simulink model "RT_Klausur_2011_A1"  (R2013a)
settings: Solver=ode45  StartTime=0.0  StopTime=10.0  RelTol=1e-3
values from neighbouring files (symbols this model uses):
  k = 1    [RT_Klausur_SS2014.m]    (also in RT_ctrl_analyse_proc.m = 5; RT_dennis_draussen.m = 50; RT_klausurvorb.m = 0.2; RT_lab_paramLead.m)
settings Model: Creator=mainster  LastModifiedBy=mainster

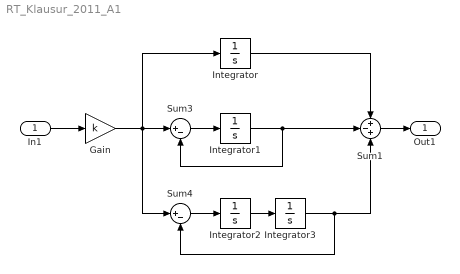
== system RT_Klausur_2011_A1 ==
  In1 : Inport
  Gain : Gain  Gain=k
  Integrator{,1..3} (4 alike) : Integrator
  Sum1 : Sum  Inputs=+-+
  Sum3 : Sum  Inputs=|+-
  Sum4 : Sum  Inputs=|+-
  Out1 : Outport
  wires:
  In1/1 -> Gain/1
  Gain/1 -> Sum4/1, Sum3/1, Integrator/1
  Sum3/1 -> Integrator1/1
  Integrator/1 -> Sum1/1
  Integrator1/1 -> Sum3/2, Sum1/2
  Sum4/1 -> Integrator2/1
  Integrator2/1 -> Integrator3/1
  Integrator3/1 -> Sum1/3, Sum4/2
  Sum1/1 -> Out1/1
